simulink model "Energy_management_controller"  (R2014a)
settings: Solver=ode45  SolverMode=SingleTasking  StartTime=0.0  StopTime=10.0  RelTol=1e-3
libraries: fuzblock x1
(part 2 of 2)

== matlab function Energy_management_controller/Energy management system for power split between FC and BAT/MATLAB Function ==
  data: u input; y output
function y = fcn(u)
 if u>=0&&u<0.05
     u=0;
%   else if u>=0.02&&u<0.07
%           u = 0.05;
%          else if u>=0.05&&u<0.12
%           u = 0.1;
%              else if u>=0.12&&u<0.17
%           u = 0.15;
               else if u>=0.05&&u<0.3
          u = 0.2;
%                 else if u>=0.22&&u<0.27
%           u = 0.25;
%                   else if u>=0.27&&u<0.32
%           u = 0.3;
%                      else if u>=0.32&&u<0.37
%           u = 0.35;
                        else if u>=0.3&&u<0.5
          u = 0.4;
%                              else if u>=0.42&&u<0.47
%           u = 0.45;
%                                 else if u>=0.47&&u<0.52
%                               u = 0.5;
%                              else if u>=0.52&&u<0.57
%                               u = 0.55;
                                 else if u>=0.5&&u<0.7
                              u = 0.6;
%                                    else if u>=0.62&&u<0.67
%                               u = 0.65;
%                                     else if u>=0.67&&u<0.72
%                               u = 0.7;
%                                       else if u>=0.72&&u<0.77
%                               u = 0.75;
%                                          else if u>=0.7&&u<0.9
%                               u = 0.8;
%                                             else if u>=0.82&&u<0.87
%                               u = 0.85;
%                                                  else if u>=0.87&&u<0.92
%                               u = 0.9;
                                                     else
                                                         u = 0.8
%                                                      end
%                                                 end
%                                              end
%                                           end
%                                         end
%                                        end
                                     end
%                                 end
%                                     end
%                                  end
                            end
%                          end
%                       end
%                     end
                    end
%                  end
%              end
%       end
 end
 
y = u;
